simulink subsystem "sensor_data_format"  (R2024a)
settings: Solver=VariableStepAuto  StartTime=0.0  StopTime=10.0  RelTol=1e-3
settings Model: Creator=gurt1  LastModifiedBy=gurt1

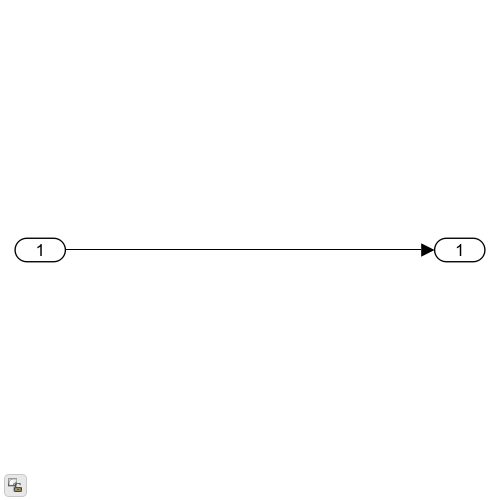
[thumbnail: Simulink's stored preview of the top-level diagram]
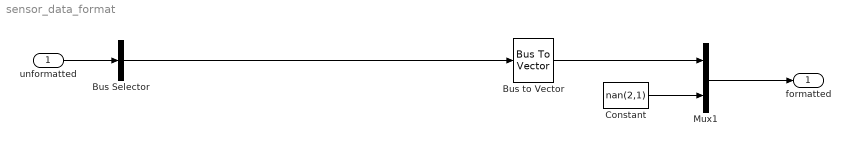
== system sensor_data_format ==
  unformatted : Inport
  Bus Selector : BusSelector  OutputSignals=att_rad,ang_rps,pos_ned_m,vel_ned_mps,alt_m,vt_kts,rho_kgmp3,flags  OutputAsBus=on
  Bus to Vector : BusToVector
  Constant : Constant  Value=nan(2,1)
  Mux1 : Mux  Inputs=2
  formatted : Outport
  wires:
  unformatted/1 -> Bus Selector/1
  Bus Selector/1 -> Bus to Vector/1
  Constant/1 -> Mux1/2
  Mux1/1 -> formatted/1
  Bus to Vector/1 -> Mux1/1
